simulink model "PaceMaker_Simulink_Model"  (R2018b)
settings: Solver=FixedStepAuto  StartTime=0.0  StopTime=inf  FixedStep=1e-3  RelTol=1e-3  EnableMultiTasking=on
undefined symbols (not defined in the file): A0, A1, D0, D1, D10, D11, D12, D13, D2, D3, D5, D6, D8, D9, PTA0, PTA1, PTA2, PTB2, PTB3, PTB9, PTC16, PTC17, PTC2, PTC4, PTD0, PTD1, PTD2, PTD3
libraries: frdmk64flib x21
(part 2 of 2)

== stateflow chart PaceMaker_Simulink_Model/System inputs /Chart1 ==
  settings: executeAtInitialization=1
  state Data
    entry:
    mode = rxdata(2);
    Lower_ratelimit =rxdata(3);
    Upper_ratelimit =rxdata(4);
    Vent_Amplitude =rxdata(5);
    Vent_PW =rxdata(6);
    At_Amplitude = rxdata(7);
    At_PW = rxdata(8);
    VRP =rxdata(9);
    ARP = rxdata(10);;
    Hysterisis =rxdata(11);
    Act_Thrs = rxdata(12);
    Maximum_sensor = rxdata(13);
    Rxn_time = rxdata(14);
    Resp_fact = rxdata(15);
    Rec_time= rxdata(16);
    %send_param();
  state INITIAL
    entry:
    Lower_ratelimit =0;
    Upper_ratelimit =0;
    Vent_Amplitude =0;
    Vent_PW =0;
    At_Amplitude = 0;
    At_PW =0;
    VRP =0;
    ARP =0;
    Hysterisis =0;
    Act_Thrs = 0;
    Maximum_sensor = 0;
    Rxn_time = 0;
    Resp_fact = 0;
    Rec_time= 0;
  state STANDBY
  state Egram
    entry:
    send_egram();
  (default) -> INITIAL
  Data -> STANDBY
  (junction 26) -> STANDBY [order 3]
  STANDBY -> (junction 26) : [status ==0]
  (junction 26) -> Data [order 1] : [rxdata(1)==1000]
  INITIAL -> STANDBY
  Egram -> (junction 26) [order 1] : [status ==0]
  (junction 26) -> Egram [order 2] : [rxdata(1)==2000]
  Egram -> Egram [order 2]
  data: mode output uint16; rxdata input uint16; status input uint8; Lower_ratelimit output uint16; Upper_ratelimit output uint16; Vent_Amplitude output uint16; Vent_PW output uint16; At_Amplitude output uint16; At_PW output uint16; VRP output uint16; ARP output uint16; Hysterisis output uint16; Act_Thrs output uint16; Maximum_sensor output uint16; Rxn_time output uint16; Resp_fact output uint16; Rec_time output uint16

== stateflow chart PaceMaker_Simulink_Model/Pacing Subsystem /AAI/AAI ==
  state Charging_C22_and_Discharging_C22
    entry:
    ATR_PACE_CTRL6=false;
    PACE_CHARGE_CTRL6=true;
    ATR_GND_CTRL6=true;
    PACE_GND_CTRL6=true;
    PACING_REF_PWM6=Atrial_Amplitude;
    redLED6=false;
    blueLED6=true;
    greenLED6=false;
    Upper_Rate_Limit;
  state Discharging_C22_and_charging_C22
    entry:
    PACE_CHARGE_CTRL6=false;
    ATR_GND_CTRL6=false;
    PACE_GND_CTRL6=true;
    ATR_PACE_CTRL6=true;
    redLED6 = false;
    greenLED6 = false;
    blueLED6 = false;
  state Inhibit_Artificial_Pace2
    entry:
    blueLED6=false;
    redLED6=false;
    greenLED6=true;
  note: Including the Refractory
      | Period after any atrial event
  (default) -> Charging_C22_and_Discharging_C22
  Charging_C22_and_Discharging_C22 -> Discharging_C22_and_charging_C22 [order 1] : [after(((60000/Lower_Rate_Limit)-Atrial_Pulse_Width-ARP_ms),msec)]
  Discharging_C22_and_charging_C22 -> Charging_C22_and_Discharging_C22 : [after(Atrial_Pulse_Width,msec)]
  Inhibit_Artificial_Pace2 -> Charging_C22_and_Discharging_C22 [order 2] : [ATR_SENSING_BOOLEAN == false]
  Charging_C22_and_Discharging_C22 -> (junction 50) [order 2] : [ATR_SENSING_BOOLEAN == true]
  Inhibit_Artificial_Pace2 -> (junction 50) [order 1] : [ATR_SENSING_BOOLEAN == true]
  (junction 50) -> Inhibit_Artificial_Pace2 : [after(ARP_ms,msec)]
  data: ATR_GND_CTRL6 output boolean; ATR_PACE_CTRL6 output boolean; PACE_CHARGE_CTRL6 output boolean; PACE_GND_CTRL6 output boolean; PACING_REF_PWM6 output uint16; Lower_Rate_Limit input uint16; Atrial_Amplitude input uint16; Atrial_Pulse_Width input uint16; ATR_SENSING_BOOLEAN input boolean; ARP_ms input uint16; blueLED6 output boolean; greenLED6 output boolean; redLED6 output boolean; Upper_Rate_Limit input uint16

== stateflow chart PaceMaker_Simulink_Model/Pacing Subsystem /AAIR/AAIR ==
  state INIT
    entry:
    rate=double(Lower_Rate_Limit);
  state Discharging_C22_and_charging_C21
    entry:
    PACE_CHARGE_CTRL8=false;
    ATR_GND_CTRL8=false;
    PACE_GND_CTRL8=true;
    ATR_PACE_CTRL8=true;
  state Charging_C22_and_Discharging_C21
    entry:
    ATR_PACE_CTRL8=false;
    PACE_CHARGE_CTRL8=true;
    ATR_GND_CTRL8=true;
    PACE_GND_CTRL8=true;
    PACING_REF_PWM8=Atrial_Amplitude;
    Upper_Rate_Limit;
  state Pace_slower
    entry:
    rate=rate-(Rate_Of_Decrease_Of_Rate)*(60/rate);
  state Pace_slower1
    entry:
    rate=rate-(Rate_Of_Increase_Of_Rate)*(60/rate);
  state Empty
    entry:
  state Inhibit_Artificial_Pace2
    entry:
    blueLED8=false;
    redLED8=false;
    greenLED8=true;
  (default) -> INIT
  (junction 67) -> Charging_C22_and_Discharging_C21 [order 1] : [ACCEL_BOOL == true]
  Discharging_C22_and_charging_C21 -> (junction 67) : [after(Atrial_Pulse_Width,msec)]
  (junction 67) -> (junction 71) [order 2] : [ACCEL_BOOL==false]
  INIT -> Charging_C22_and_Discharging_C21
  Pace_slower -> Charging_C22_and_Discharging_C21
  (junction 71) -> Pace_slower [order 1] : [rate > Lower_Rate_Limit]
  (junction 71) -> Charging_C22_and_Discharging_C21 [order 2] : [rate <= Lower_Rate_Limit]
  Pace_slower1 -> Discharging_C22_and_charging_C21 : [after(((60000/rate)-Atrial_Pulse_Width),msec)]
  (junction 80) -> Discharging_C22_and_charging_C21 : [after(((60000/rate)-Atrial_Pulse_Width),msec)]
  (junction 75) -> Pace_slower1 [order 1] : [rate < Max_Sensor_Rate]
  (junction 75) -> (junction 80) [order 2] : [rate >= Max_Sensor_Rate]
  Inhibit_Artificial_Pace2 -> Charging_C22_and_Discharging_C21 : [ATR_SENSING_BOOLEAN == false]
  Empty -> (junction 75) [order 2] : [(ATR_SENSING_BOOLEAN == false) && (ACCEL_BOOL==true)]
  Empty -> Discharging_C22_and_charging_C21 [order 3] : [after(((60000/rate)-Atrial_Pulse_Width-ARP_ms),msec)]
  Charging_C22_and_Discharging_C21 -> Empty : [after(ARP_ms,msec)]
  Empty -> Inhibit_Artificial_Pace2 [order 1] : [ATR_SENSING_BOOLEAN == true]
  data: Lower_Rate_Limit input uint16; PACE_CHARGE_CTRL8 output boolean; PACE_GND_CTRL8 output boolean; PACING_REF_PWM8 output uint16; ATR_GND_CTRL8 output boolean; ATR_PACE_CTRL8 output boolean; Atrial_Amplitude input uint16; Atrial_Pulse_Width input uint16; ATR_SENSING_BOOLEAN input boolean; ACCEL_BOOL input boolean; Max_Sensor_Rate input uint16; Rate_Of_Increase_Of_Rate input double; Upper_Rate_Limit input uint16; ARP_ms input uint16; Reaction_Time input; rate local double; blueLED8 output boolean; greenLED8 output boolean; redLED8 output boolean; Rate_Of_Decrease_Of_Rate input double

== stateflow chart PaceMaker_Simulink_Model/Pacing Subsystem /VVI /VVI ==
  state Charging_C22_and_Discharging_C22
    entry:
    VENT_PACE_CTRL5=false;
    PACE_CHARGE_CTRL5=true;
    VENT_GND_CTRL5=true;
    PACE_GND_CTRL5=true;
    PACING_REF_PWM5=Ventricular_Amplitude;
    redLED5=false;
    blueLED5=true;
    greenLED5=false;
    Upper_Rate_Limit;
  state Discharging_C22_and_charging_C22
    entry:
    PACE_CHARGE_CTRL5=false;
    VENT_GND_CTRL5=false;
    PACE_GND_CTRL5=true;
    VENT_PACE_CTRL5=true;
    redLED5 = false;
    greenLED5 = false;
    blueLED5 = false;
  state Inhibit_Artificial_Pace2
    entry:
    blueLED5=false;
    redLED5=false;
    greenLED5=true;
  note: Including the Refractory Period
      | after any ventricular event
  (default) -> Charging_C22_and_Discharging_C22
  Charging_C22_and_Discharging_C22 -> Discharging_C22_and_charging_C22 [order 1] : [after(((60000/Lower_Rate_Limit)-Ventricular_Pulse_Width-VRP_ms),msec)]
  Discharging_C22_and_charging_C22 -> Charging_C22_and_Discharging_C22 : [after(Ventricular_Pulse_Width,msec)]
  Inhibit_Artificial_Pace2 -> Charging_C22_and_Discharging_C22 [order 2] : [VENT_SENSING_BOOLEAN == false]
  Charging_C22_and_Discharging_C22 -> (junction 82) [order 2] : [VENT_SENSING_BOOLEAN == true]
  Inhibit_Artificial_Pace2 -> (junction 82) [order 1] : [VENT_SENSING_BOOLEAN == true]
  (junction 82) -> Inhibit_Artificial_Pace2 : [after(VRP_ms,msec)]
  data: Lower_Rate_Limit input uint16; PACE_CHARGE_CTRL5 output boolean; PACE_GND_CTRL5 output boolean; PACING_REF_PWM5 output uint16; VENT_GND_CTRL5 output boolean; VENT_PACE_CTRL5 output boolean; Ventricular_Amplitude input uint16; Ventricular_Pulse_Width input uint16; VENT_SENSING_BOOLEAN input boolean; VRP_ms input uint16; blueLED5 output boolean; greenLED5 output boolean; redLED5 output boolean; Upper_Rate_Limit input uint16

== matlab function PaceMaker_Simulink_Model/Accelerometer subsysterm /MATLAB Function ==
  data: Activity_Threshold input double; ACCEL_BOOL output boolean; Accel_Mag input double
function ACCEL_BOOL = fcn(Activity_Threshold, Accel_Mag)

if Accel_Mag > Activity_Threshold
    ACCEL_BOOL=true;
else
    ACCEL_BOOL=false;
end

== stateflow chart PaceMaker_Simulink_Model/Pacing Subsystem /VVIR/VVIR ==
  state INIT
    entry:
    rate=double(Lower_Rate_Limit);
  state Discharging_C22_and_charging_C21
    entry:
    PACE_CHARGE_CTRL7=false;
    VENT_GND_CTRL7=false;
    PACE_GND_CTRL7=true;
    VENT_PACE_CTRL7=true;
  state Charging_C22_and_Discharging_C21
    entry:
    VENT_PACE_CTRL7=false;
    PACE_CHARGE_CTRL7=true;
    VENT_GND_CTRL7=true;
    PACE_GND_CTRL7=true;
    PACING_REF_PWM7=Ventricular_Amplitude;
    Upper_Rate_Limit;
  state Pace_slower
    entry:
    rate=rate-(Rate_Of_Decrease_Of_Rate)*(60/rate);
  state Pace_slower1
    entry:
    rate=rate-(Rate_Of_Increase_Of_Rate)*(60/rate);
  state Empty
    entry:
  state Inhibit_Artificial_Pace2
    entry:
    blueLED7=false;
    redLED7=false;
    greenLED7=true;
  (default) -> INIT
  (junction 67) -> Charging_C22_and_Discharging_C21 [order 1] : [ACCEL_BOOL == true]
  Discharging_C22_and_charging_C21 -> (junction 67) : [after(Ventricular_Pulse_Width,msec)]
  (junction 67) -> (junction 71) [order 2] : [ACCEL_BOOL==false]
  INIT -> Charging_C22_and_Discharging_C21
  Pace_slower -> Charging_C22_and_Discharging_C21
  (junction 71) -> Pace_slower [order 1] : [rate > Lower_Rate_Limit]
  (junction 71) -> Charging_C22_and_Discharging_C21 [order 2] : [rate <= Lower_Rate_Limit]
  Pace_slower1 -> Discharging_C22_and_charging_C21 : [after(((60000/rate)-Ventricular_Pulse_Width),msec)]
  (junction 75) -> Pace_slower1 [order 1] : [rate < Max_Sensor_Rate]
  Empty -> (junction 75) [order 2] : [(VENT_SENSING_BOOLEAN == false) && (ACCEL_BOOL==true)]
  (junction 75) -> (junction 80) [order 2] : [rate >= Max_Sensor_Rate]
  Inhibit_Artificial_Pace2 -> Charging_C22_and_Discharging_C21 : [VENT_SENSING_BOOLEAN == false]
  Empty -> Discharging_C22_and_charging_C21 [order 3] : [after(((60000/rate)-Ventricular_Pulse_Width-VRP_ms),msec)]
  (junction 80) -> Discharging_C22_and_charging_C21 : [after(((60000/rate)-Ventricular_Pulse_Width),msec)]
  Charging_C22_and_Discharging_C21 -> Empty : [after(VRP_ms,msec)]
  Empty -> Inhibit_Artificial_Pace2 [order 1] : [VENT_SENSING_BOOLEAN == true]
  data: Lower_Rate_Limit input uint16; PACE_CHARGE_CTRL7 output boolean; PACE_GND_CTRL7 output boolean; PACING_REF_PWM7 output uint16; VENT_GND_CTRL7 output boolean; VENT_PACE_CTRL7 output boolean; Ventricular_Amplitude input uint16; Ventricular_Pulse_Width input uint16; VENT_SENSING_BOOLEAN input boolean; ACCEL_BOOL input boolean; Max_Sensor_Rate input uint16; Rate_Of_Increase_Of_Rate input double; Upper_Rate_Limit input uint16; VRP_ms input uint16; Reaction_Time input; rate local double; blueLED7 output boolean; greenLED7 output boolean; redLED7 output boolean; Rate_Of_Decrease_Of_Rate input double

== stateflow chart PaceMaker_Simulink_Model/Pacing Subsystem /AOOR/AOOR ==
  note: - Using local variable "rate" to control
      | increasing/decreasing pulsing rate
      | - Initializing "rate" to the Lower_Rate_Limit
  state INITIAL
    entry:
    rate=double(Lower_Rate_Limit);
    time=0;
  state Discharging_C22_and_charging_C21
    entry:
    PACE_CHARGE_CTRL4=false;
    ATR_GND_CTRL4=false;
    PACE_GND_CTRL4=true;
    ATR_PACE_CTRL4=true;
    redLED4=true;
    greenLED4=false;
  state Charging_C22_and_Discharging_C21
    entry:
    ATR_PACE_CTRL4=false;
    PACE_CHARGE_CTRL4=true;
    ATR_GND_CTRL4=true;
    PACE_GND_CTRL4=true;
    PACING_REF_PWM4=Atrial_Amplitude;
    redLED4=false;
    greenLED4=false;
  state Pace_slower
    entry:
    rate=rate-(Rate_Of_Decrease_Of_Rate)*(60/rate);
    redLED4=false;
    greenLED4=true;
    if rate<Lower_Rate_Limit
    rate=double(60);
    else
    rate=rate;
    end
  state Pace_faster
    entry:
    rate=rate+(Rate_Of_Increase_Of_Rate)*double(60/rate);
    redLED4=false;
    greenLED4=false;
    if rate>Max_Sensor_Rate
    rate=double(120);
    else
    rate=rate;
    end
  (default) -> INITIAL
  Charging_C22_and_Discharging_C21 -> Discharging_C22_and_charging_C21 [order 1] : [after(((60000/rate)-Atrial_Pulse_Width-10),msec)]{time=time+(60/rate)}
  INITIAL -> Charging_C22_and_Discharging_C21
  Discharging_C22_and_charging_C21 -> (junction 164) : [after(Atrial_Pulse_Width,msec)]
  (junction 164) -> Charging_C22_and_Discharging_C21 [order 2] : [ACCEL_BOOL == true]
  (junction 164) -> (junction 165) [order 1] : [ACCEL_BOOL == false]{time=0}
  Pace_slower -> Charging_C22_and_Discharging_C21 : [after(10,msec)]
  (junction 165) -> Pace_slower [order 2] : [rate > Lower_Rate_Limit]
  (junction 165) -> Charging_C22_and_Discharging_C21 [order 1] : [rate <= Lower_Rate_Limit]
  Pace_faster -> Discharging_C22_and_charging_C21 : [after(((60000/rate)-Atrial_Pulse_Width),msec)]
  (junction 162) -> Discharging_C22_and_charging_C21 : [after(((60000/rate)-Atrial_Pulse_Width),msec)]
  Charging_C22_and_Discharging_C21 -> (junction 163) [order 2] : [(time>Reaction_Time) && (ACCEL_BOOL == true)]
  (junction 163) -> Pace_faster [order 2] : [rate < Max_Sensor_Rate]
  (junction 163) -> (junction 162) [order 1] : [rate >= Max_Sensor_Rate]
  data: PACE_CHARGE_CTRL4 output boolean; PACE_GND_CTRL4 output boolean; PACING_REF_PWM4 output uint16; ATR_GND_CTRL4 output boolean; ATR_PACE_CTRL4 output boolean; Atrial_Amplitude input uint16; Max_Sensor_Rate input uint16; ACCEL_BOOL input boolean; rate local double; greenLED4 output boolean; redLED4 output boolean; Lower_Rate_Limit input uint16; Atrial_Pulse_Width input uint16; Rate_Of_Decrease_Of_Rate input double; Rate_Of_Increase_Of_Rate input double; time local double; Reaction_Time input uint16

== matlab function PaceMaker_Simulink_Model/Pacing Subsystem /MATLAB Function ==
  data: vector input; PCC output; Flag_Number input
function PCC = fcn(vector,Flag_Number)
PCC = vector(Flag_Number);

== matlab function PaceMaker_Simulink_Model/Pacing Subsystem /MATLAB Function1 ==
  data: vector input; PRP output; Flag_Number input
function PRP = fcn(vector,Flag_Number)
PRP = vector(Flag_Number);

== matlab function PaceMaker_Simulink_Model/Pacing Subsystem /MATLAB Function2 ==
  data: vector input; RL output; Flag_Number input
function RL = fcn(vector,Flag_Number)
RL = vector(Flag_Number);

== matlab function PaceMaker_Simulink_Model/Pacing Subsystem /MATLAB Function3 ==
  data: vector input; AGC output; Flag_Number input
function AGC = fcn(vector,Flag_Number)

switch Flag_Number
    case 2
        AGC=vector(1);
    case 4
        AGC=vector(2);
    case 6
        AGC=vector(3);
    case 8
        AGC=vector(4);
    otherwise
        AGC=false;
end

== matlab function PaceMaker_Simulink_Model/Pacing Subsystem /MATLAB Function4 ==
  data: vector input; APC output; Flag_Number input
function APC = fcn(vector,Flag_Number)

switch Flag_Number
    case 2
        APC=vector(1);
    case 4
        APC=vector(2);
    case 6
        APC=vector(3);
    case 8
        APC=vector(4);
    otherwise
        APC=false;
end

== matlab function PaceMaker_Simulink_Model/Pacing Subsystem /MATLAB Function5 ==
  data: vector input; GL output; Flag_Number input
function GL = fcn(vector,Flag_Number)

switch Flag_Number
    case 3
        GL=vector(1);
    case 4
        GL=vector(2);
    case 5
        GL=vector(3);
    case 6
        GL=vector(4);
    case 7
        GL=vector(5);
    case 8
        GL=vector(6);
    otherwise
        GL=false;
end

== matlab function PaceMaker_Simulink_Model/Pacing Subsystem /MATLAB Function6 ==
  data: vector input; PGC output; Flag_Number input
function PGC = fcn(vector,Flag_Number)
PGC = vector(Flag_Number);

== matlab function PaceMaker_Simulink_Model/Pacing Subsystem /MATLAB Function7 ==
  data: vector input; VGC output; Flag_Number input
function VGC = fcn(vector,Flag_Number)

switch Flag_Number
    case 1
        VGC=vector(1);
    case 3
        VGC=vector(2);
    case 5
        VGC=vector(3);
    case 7
        VGC=vector(4);
    otherwise
        VGC=false;
end

== matlab function PaceMaker_Simulink_Model/Pacing Subsystem /MATLAB Function8 ==
  data: vector input; VPC output; Flag_Number input
function VPC = fcn(vector,Flag_Number)

switch Flag_Number
    case 1
        VPC=vector(1);
    case 3
        VPC=vector(2);
    case 5
        VPC=vector(3);
    case 7
        VPC=vector(4);
    otherwise
        VPC=false;
end

== matlab function PaceMaker_Simulink_Model/Pacing Subsystem /MATLAB Function9 ==
  data: vector input; BL output; Flag_Number input
function BL = fcn(vector,Flag_Number)

switch Flag_Number
    case 5
        BL=vector(1);
    case 6
        BL=vector(2);
    case 7
        BL=vector(3);
    case 8
        BL=vector(4);
    otherwise
        BL=false;
end

== matlab function PaceMaker_Simulink_Model/Sensing Subsystem/MATLAB Function ==
  data: vector input; Front_End_Ctrl output; Flag_Number input
function Front_End_Ctrl = fcn(vector,Flag_Number)

switch Flag_Number
    case 5
        Front_End_Ctrl=vector(1);
    case 6
        Front_End_Ctrl=vector(2);
    case 7
        Front_End_Ctrl=vector(1);
    case 8
        Front_End_Ctrl=vector(2);
    otherwise
        Front_End_Ctrl=false;
end
